simulink model "Sensitivity_Analysis"  (R2023a)
settings: Solver=VariableStepAuto  StartTime=0.0  StopTime=10.0  RelTol=1e-3
PreLoadFcn:
  | g = 9.086;
model workspace (MAT data in the model file):
  I1 = 6016241.326
  I2 = 7399466.245
  I3 = 689920.7492
  I4 = 52.42660048
  I5 = 4.678936735
  Ms = 2849.727161
  chi0 = 0.1
  g = 9.806
  r1 = 7.004079989
  r2 = 17.29333946
  r3 = 22.26700704
  r4 = 24.99999999
  r5 = 25
  rho = 1045.639438
  w = 0.585459507
  z1 = -5.999999958
  z2 = 3.361582194
  z3 = 4.429855921
  z4 = -5.999999987
  z5 = -5.999999987
values from neighbouring files (symbols this model uses):
  I6 = x(17)    [errorFcn_10coils.m]    (also in errorFcn_6coils.m)
  r6 = x(19)    [errorFcn_10coils.m]    (also in errorFcn_6coils.m)
  z6 = x(18)    [errorFcn_10coils.m]    (also in errorFcn_6coils.m)
settings Model: Creator=hutianyang  LastModifiedBy=hutianyang

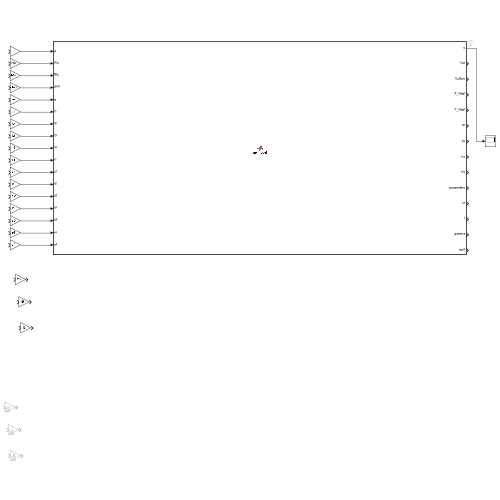
[thumbnail: Simulink's stored preview of the top-level diagram]
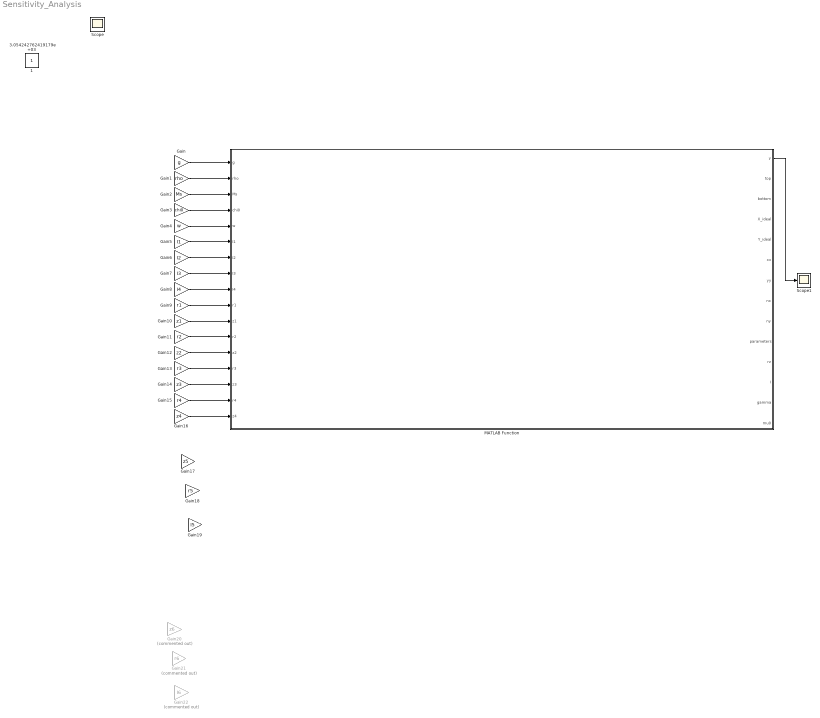
== system Sensitivity_Analysis ==
  Gain : Gain  Gain=g
  Gain1 : Gain  Gain=rho
  Gain10 : Gain  Gain=z1
  Gain11 : Gain  Gain=r2
  Gain12 : Gain  Gain=z2
  Gain13 : Gain  Gain=r3
  Gain14 : Gain  Gain=z3
  Gain15 : Gain  Gain=r4
  Gain16 : Gain  Gain=z4
  Gain17 : Gain  Gain=z5
  Gain18 : Gain  Gain=r5
  Gain19 : Gain  Gain=I5
  Gain2 : Gain  Gain=Ms
  Gain20 : Gain  Commented=on  Gain=z6
  Gain21 : Gain  Commented=on  Gain=r6
  Gain22 : Gain  Commented=on  Gain=I6
  Gain3 : Gain  Gain=chi0
  Gain4 : Gain  Gain=w
  Gain5 : Gain  Gain=I1
  Gain6 : Gain  Gain=I2
  Gain7 : Gain  Gain=I3
  Gain8 : Gain  Gain=I4
  Gain9 : Gain  Gain=r1
  MATLAB Function : MATLAB Function  TreatAsAtomicUnit=on
  Scope1 : Scope
  1 : Constant  IOType=siggen
  3.054242762419179e+03 : Constant  IOType=siggen
  Scope : Scope
  wires:
  MATLAB Function/1(y) -> Scope1/1
  Gain1/1 -> MATLAB Function/2(rho)
  Gain/1 -> MATLAB Function/1(g)
  Gain2/1 -> MATLAB Function/3(Ms)
  Gain3/1 -> MATLAB Function/4(chi0)
  Gain4/1 -> MATLAB Function/5(w)
  Gain5/1 -> MATLAB Function/6(I1)
  Gain6/1 -> MATLAB Function/7(I2)
  Gain7/1 -> MATLAB Function/8(I3)
  Gain8/1 -> MATLAB Function/9(I4)
  Gain9/1 -> MATLAB Function/10(r1)
  Gain10/1 -> MATLAB Function/11(z1)
  Gain11/1 -> MATLAB Function/12(r2)
  Gain12/1 -> MATLAB Function/13(z2)
  Gain13/1 -> MATLAB Function/14(r3)
  Gain14/1 -> MATLAB Function/15(z3)
  Gain15/1 -> MATLAB Function/16(r4)
  Gain16/1 -> MATLAB Function/17(z4)

== matlab function Sensitivity_Analysis/MATLAB Function ==
  data: g input; y output; rho input; Ms input; chi0 input; w input; I1 input; I2 input; I3 input; I4 input; r1 input; z1 input; r2 input; z2 input; r3 input; z3 input; r4 input; z4 input; top output; bottom output; X_ideal output; Y_ideal output; xx output; yy output; nx output; ny output; parameters output; rz output; I output; gamma output; mu0 output
function [y,top,bottom,X_ideal,Y_ideal,xx,yy,nx,ny,parameters,rz,I,gamma,mu0] = mymodel(g,rho,Ms,chi0,w,I1,I2,I3,I4,r1,z1,r2,z2,r3,z3,r4,z4)
%MYMODEL This is the math model of spherical mirror used for sensitivity analysis
%--------------------------------------------------------------------------------------
%   Inputs: 
%          g                    Gravitational acceleration       [m/s^2]
%          rho                  Density of ferrofluid            [kg/m^3]
%          Ms                   Saturation magnetization         [A/m]
%          chi0                 Initial Magenetic susceptibility
%          w                    Angular velocity of disk         [rad/s]
%          [I1, I2, I3, I4]     Current inside coils             [A]
%          [r1 z1;
%           r2 z2;
%           r3 z3;
%           r4 z4]              Coil positions in 2D             [m]

%---------------------------------------------------------------------------------------
%   Output: error is maximum of the absolute value of deviation(at each point along the spherical 
%           mirror surface) from the ideal surface
%---------------------------------------------------------------------------------------
%   Date:   10-31-2023
%%

mu0              = 4*pi*1e-7;               % Vaccum Pemeability [N/A^2]
gamma            = 3*chi0/Ms;
I                = [I1;I2;I3;I4];           % Current inside each coil [A]
rz               = [r1,z1;    
                    r2,z2;
                    r3,z3;
                    r4,z4];                 % Positions of coils [m]
parameters       = [g;mu0;rho;Ms;gamma];
N_count          = 91;
r_flat           = 15;
step             = 0.0001;
[xx, yy, nx, ny] = surface_params(r_flat, N_count, step); 
X_ideal          = zeros(1, N_count);
Y_ideal          = zeros(1, N_count);
top              = massForcePotential(w,xx',yy',I,rz,parameters) - massForcePotential(w,X_ideal',Y_ideal',I,rz,parameters);
bottom           = 1/(2*step) * (massForcePotential(w,(xx+step*nx)',(yy+step*ny)',I,rz,parameters) - massForcePotential(w,(xx-step*nx)',(yy-step*ny)',I,rz,parameters));
y                = max(abs((top./bottom)));
end
